simulink library "seriallib"  (Simulink 5.0)
undefined symbols (not defined in the file or in its folder): mbaseserialmask, mmodemcontrol, mquamask, mrs232
libraries: xpclib x193, vxlib x36, simulink x4
(part 1 of 3)
settings Model: Creator=gweast  LastModifiedBy=gweast

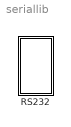
== system seriallib ==
  RS232 : Subsystem

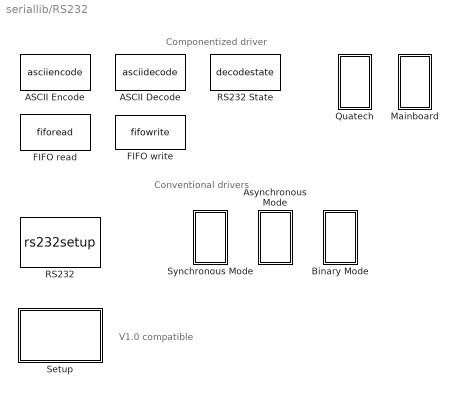
== system seriallib/RS232 ==
  note: Conventional drivers
  note: Componentized driver
  note: V1.0 compatible
  "ASCII Decode " : S-Function  FunctionName=asciidecode  Parameters=format, nvars, varids  mask(Asynchronous FIFO Block: reader){format=%d\r, nvars=1, vartypes={ }}
      mask prompts: format "Format string:"; nvars "Number of variables:"; vartypes "Variable types:"
      mask help: FIFO read
      mask init:
      | [ maskdisplay, varids, format ] = masciidecode( 2, format, nvars, vartypes, 1 );
      | set_param( gcb, 'MaskDisplay', maskdisplay );
      mask Help: helpview(fullfile(docroot, 'mapfiles', 'xpc.map'), 'Quatech_ASCII_Decode')
      mask Display: disp( 'ASCII\nDecode');port_label('input',1,'D');port_label('output',1,'1');
  "ASCII Encode " : S-Function  FunctionName=asciiencode  Parameters=format, maxlength, nvars, varids  mask(Ascii Encode){format=%d\r, nvars=1, maxlength=128, vartypes={ 'double' }}
      mask prompts: format "Format string:"; nvars "Number of variables:"; maxlength "Max output string length:"; vartypes "Variable types:"
      mask help: Ascii Encode -- encode input variables as ascii for RS232.
      mask init:
      | [ maskdisplay, varids, format ] = masciidecode( 2, format, nvars, vartypes, 2 );
      | set_param( gcb, 'MaskDisplay', maskdisplay );
      mask Help: helpview(fullfile(docroot, 'mapfiles', 'xpc.map'), 'Quatech_ASCII_Encode')
      mask Display: disp( 'ASCII\nEncode');port_label('output',1,'D');port_label('input',1,'1');
  Asynchronous Mode : Subsystem
  Binary Mode : Subsystem
  "FIFO read " : S-Function  FunctionName=fiforead  Parameters=maxsize, minsize, usedelimiter, delimiter, outputtype, sampletime, enable, enableout  mask(Asynchronous FIFO Block: reader){maxsize=1024, minsize=1, usedelimiter=on, delimiter=13, outputtype=8 bit uint null terminated, enable=off, enableout=off, sampletime=0.001}
      mask prompts: maxsize "Maximum read size:"; minsize "Minimum read size:"; usedelimiter "Read to delimiter:"; outputtype "Output vector type:"; enable "Max and Min read size ports:"; enableout "Enable passthrough:"
      mask help: FIFO read
      mask init:
      | maskdisplay = mfiforw( enable, enableout, 2 );
      | set_param( gcb, 'MaskDisplay', maskdisplay );
      mask Help: helpview(fullfile(docroot, 'mapfiles', 'xpc.map'), 'Quatech_FIFO_Read')
      mask StyleString: edit,edit,checkbox,edit,popup(count+32 bit int|count+32 bit uint|count+16 bit int|count+16 bit uint|8 bit int null terminated|8 bit uint null terminated),checkbox,checkbox,edit
      mask Display: disp( 'FIFO\nRead');port_label('output',1,'D');port_label('input',1,'F');
  "FIFO write " : S-Function  FunctionName=fifowrite  Parameters=size, inputtype, sampletime, present  mask(Asynchronous FIFO Block: writer){size=1024, inputtype=8 bit uint null terminated, present=off, sampletime=-1}
      mask prompts: inputtype "Input vector type:"; present "Data present output:"
      mask help: FIFO write
      mask init:
      | maskdisplay = mfiforw( present, 0, 1 );
      | set_param(gcb,'MaskDisplay',maskdisplay);
      mask Help: helpview(fullfile(docroot, 'mapfiles', 'xpc.map'), 'Quatech_FIFO_Write')
      mask StyleString: edit,popup(count+32 bit int|count+32 bit uint|count+16 bit int|count+16 bit uint|8 bit int null terminated|8 bit uint null terminated),checkbox,edit
      mask Display: disp( 'FIFO\nwrite');port_label('input',1,'D');port_label('output', 1, 'F');
  Mainboard : Subsystem
  Quatech : Subsystem
  "RS232 " : S-Function  InitFcn=mrs232(0);  FunctionName=rs232setup  Parameters=port, baud, dbits, sbits, parity, prot, sbuf, rbuf, 0, istr, iack, iackto, tstr, tack, tackto, initinfo, initackinfo, terminfo, termackinfo  mask(rs232setup){port=COM1, baud=9600, dbits=8, sbits=1, parity=None, prot=None, sbuf=1024, rbuf=1024, initstruct=[], termstruct=[]}
      mask prompts: baud "Baud rate:"; dbits "Number of data bits:"; sbits "Number of stop bits:"; prot "Protocol:"; sbuf "Send buffer size:"; rbuf "Receive buffer size:"; initstruct "Initialization command structure:"; termstruct "Termination command structure:"
      mask help:
      | RS-232
      | Mainboard
      | Setup
      mask init:
      | dmy = '';
      | [istr,iack,dmy,maskdisplay,maskdescription,dmy,dmy,dmy,dmy,initinfo,initackinfo,iackto]=mrs232(2,initstruct,4);
      | [tstr,tack,dmy,maskdisplay,maskdescription,dmy,dmy,dmy,dmy,terminfo,termackinfo,tackto]=mrs232(1,termstruct,4);
      | set_param(gcb,'MaskDisplay',maskdisplay);
      | set_param(gcb,'MaskDescription',maskdescription);
      mask Help: helpview(fullfile(docroot, 'mapfiles', 'xpc.map'), 'RS232_RS232')
      mask StyleString: popup(COM1|COM2|COM3|COM4),popup(115200|57600|38400|19200|9600|4800|2400|1200|600|300|110),popup(8|7),popup(1|2),popup(None|Odd|Even),popup(None|XOn XOff),edit,edit,edit,edit
      mask Display: disp('RS-232\nMainboard\nSetup');
  RS232 State : S-Function  FunctionName=decodestate  Parameters=overrun, parity, frame, breakint, count  mask(RS232 State){overrun=on, parity=on, frame=off, breakint=off}
      mask prompts: overrun "Overrun error output:"; parity "Parity error output"; frame "Framing error output"; breakint "Break interrupt output"
      mask help: RS232 State
      mask init:
      | count = 0;
      | [maskdisplay, count] = mdecodestate( overrun, parity, frame, breakint );
      | set_param( gcb, 'MaskDisplay', maskdisplay );
      mask Help: helpview(fullfile(docroot, 'mapfiles', 'xpc.map'), 'Quatech_State')
      mask Display: disp('RS232\nState');port_label('input',1,'D');port_label('output',1,'D');port_label('output',2,'O');port_label('output',3,'P');
  "Setup " : Subsystem  mask(rs232setup){port=COM2, baudrate=115200, databit=8, stopbit=1, parity=None, protocol=None, sendbuf=1024, recbuf=1024}
      mask prompts: baudrate "Baud rate:"; databit "Number of data bits:"; stopbit "Number of stop bits:"; sendbuf "Send buffer size:"; recbuf "Receive buffer size:"
      mask Help: helpview(fullfile(docroot,'mapfiles','xpc.map'),'RS232_Setup');
      mask StyleString: popup(COM1|COM2|COM3|COM4),popup(115200|57600|38400|19200|9600|4800|2400|1200|300|110),popup(8|7|6|5),popup(1|2),popup(None|Odd|Even),popup(None|XOnXOff|RTSCTS|DTRDSR),edit,edit
      mask Display: disp('RS232\nMainboard\nSetup');
  Synchronous Mode : Subsystem

== system seriallib/RS232/Asynchronous Mode ==
  note: V1.0 compatible
  "RS232 " : S-Function  FunctionName=rs232send  Parameters=port, inStr, inport, numinports, formatsendinfo, ts, waitarg  mask(rs232send){port=COM1, blockvar=[], ts=0.1}
      mask prompts: blockvar "Message struct name:"; ts "Sample time:"
      mask help:
      | RS-232
      | Mainboard
      | Send
      mask init:
      | inStr = '';
      | outStr = '';
      | [inStr,outStr,dtypes,maskdisplay,maskdescription,inport,outport, numinports, numoutports, formatsendinfo, formatrecinfo, waitarg] = mrs232 (1, blockvar, 2);
      | set_param(gcb,'MaskDisplay',maskdisplay);
      | set_param(gcb,'MaskDescription',maskdescription);
      mask Help: helpview(fullfile(docroot, 'mapfiles', 'xpc.map'), 'RS232_Asynchronous-Mode_RS232')
      mask StyleString: popup(COM1|COM2|COM3|COM4),edit,edit
      mask Display: disp('RS-232\nMainboard\nSend');
  RS232 1 : S-Function  FunctionName=rs232rec  Parameters=port, outStr, outport, numoutports, formatrecinfo, dtypes, ts, numeom  mask(rs232rec){port=COM1, blockvar=[], ts=0.1}
      mask prompts: blockvar "Message struct name:"; ts "Sample time:"
      mask help:
      | RS-232
      | Mainboard
      | Receive
      mask init:
      | inStr = '';
      | outStr = '';
      | [inStr,outStr,dtypes,maskdisplay,maskdescription,inport,outport, numinports, numoutports, formatsendinfo, formatrecinfo, waitarg, numeom] = mrs232 (1, blockvar, 1);
      | 
      | 
      | set_param(gcb,'MaskDisplay',maskdisplay);
      | set_param(gcb,'MaskDescription',maskdescription);
      mask Help: helpview(fullfile(docroot, 'mapfiles', 'xpc.map'), 'RS232_Asynchronous-Mode_RS232-1')
      mask StyleString: popup(COM1|COM2|COM3|COM4),edit,edit
      mask Display: disp('RS-232\nMainboard\nReceive');
  "Receive " : Subsystem  mask(rs232rec){port=COM2, formatrec='start,%f,stop;', numb=1, ts=0.01}
      mask prompts: formatrec "Receive format:"; numb "Number of end-of-message characters:"; ts "Sample time:"
      mask Help: helpview(fullfile(docroot, 'mapfiles', 'xpc.map'), 'RS232_Asynchronous-Mode_Receive')
      mask StyleString: popup(COM1|COM2|COM3|COM4),edit,edit,edit
      mask Display: disp('RS232\nMainboard\nReceive');
  "Send " : Subsystem  mask(rs232send){port=COM2, formatsend='start,%f,stop;', wait=off, ts=0.01}
      mask prompts: formatsend "Send format:"; wait "Wait until message is transmitted"; ts "Sample time:"
      mask Help: helpview(fullfile(docroot, 'mapfiles', 'xpc.map'), 'RS232_Asynchronous-Mode_Send')
      mask StyleString: popup(COM1|COM2|COM3|COM4),edit,checkbox,edit
      mask Display: disp('RS232\nMainboard\nSend');

== system seriallib/RS232/Binary Mode ==
  Pack : xpclib/UDP/Pack  datatypes={'double'}  byteAlign=1
  RS232 Binary Receive : S-Function  FunctionName=rs232brec  Parameters=port,width,samptime  mask(rs232brec){port=COM1, width=1, samptime=-1}
      mask prompts: port "COM port:"; width "Maximum width per packet:"; samptime "Sample time:"
      mask Help: helpview(fullfile(docroot, 'mapfiles', 'xpc.map'), 'RS232_Binary-Mode_RS232-Binary-Receive')
      mask StyleString: popup(COM1|COM2|COM3|COM4),edit,edit
      mask Display: port_label('input',  1, 'Length');port_label('input',  2, 'Enable');port_label('output', 1, 'Done');port_label('output', 2, 'Data');disp(sprintf('RS232 Receive\nCOM%d', port));
  RS232 Binary Send : S-Function  FunctionName=rs232bsend  Parameters=port,width,samptime  mask(rs232bsend){port=COM1, width=1, samptime=-1}
      mask prompts: port "COM port:"; width "Maximum width per packet:"; samptime "Sample time:"
      mask Help: helpview(fullfile(docroot, 'mapfiles', 'xpc.map'), 'RS232_Binary-Mode_RS232-Binary-Send')
      mask StyleString: popup(COM1|COM2|COM3|COM4),edit,edit
      mask Display: disp(sprintf('RS232 Send\nCOM%d', port));
  Unpack : xpclib/UDP/Unpack  dimensions={[1]}  datatypes={'double'}  byteAlign=1

== system seriallib/RS232/Mainboard ==
  Baseboard Serial : Subsystem  InitFcn=mbaseserialmask(4,2)  TreatAsAtomicUnit=on  mask(Baseboard RS232 Send Receive){group=Board Setup, port=1, irqnum=4, saddr1=0x3f8, saddr2=0x3e8, config=Com1/Com3, baud1=115200, parity1=None, ndata1=8, nstop1=1, fifomode1=16 deep, rlevel1=half full, automode1=on, xmtfifosize1=1024, xmtdatatype1=8 bit uint null terminated, rcvfifosize1=1024, rcvmaxread1=1024, rcvminread1=1, rcvusedelim1=on, rcvdelim1=13, rcvdatatype1=count+16 bit uint, rcvsampletime1=-1, baud2=115200, parity2=None, ndata2=8, nstop2=1, fifomode2=16 deep, rlevel2=half full, automode2=off, xmtfifosize2=1024, xmtdatatype2=8 bit uint null terminated, rcvfifosize2=1024, rcvmaxread2=1024, rcvminread2=1, rcvusedelim2=on, rcvdelim2=13, rcvdatatype2=count+16 bit uint, rcvsampletime2=-1}
      mask prompts: group "Parameter group:"; port "Port to modify:"; irqnum "IRQ number:"; saddr1 "First port address:"; saddr2 "Second port address:"; config "Configuration:"; baud1 "Baud rate:"; parity1 "Parity:"; ndata1 "Data bits:"; nstop1 "Stop bits:"; fifomode1 "Hardware fifo size:"; rlevel1 "Receive fifo interrupt level:"; automode1 "Auto RTS/CTS:"; xmtfifosize1 "Transmit software fifo size:"; xmtdatatype1 "Transmit fifo data type:"; rcvfifosize1 "Receive software fifo size:"; rcvmaxread1 "Receive maximum read:"; rcvminread1 "Receive minimum read:"; rcvusedelim1 "Read to delimiter:"; rcvdelim1 "Delimiter:"; rcvdatatype1 "Receive data type:"; rcvsampletime1 "Receive SampleTime:"; baud2 "Baud rate:"; parity2 "Parity:"; ndata2 "Data bits:"; nstop2 "Stop bits:"; fifomode2 "Hardware fifo size:"; rlevel2 "Receive fifo interrupt level:"; automode2 "Auto RTS/CTS:"; xmtfifosize2 "Transmit software fifo size:"; xmtdatatype2 "Transmit fifo data type:"; rcvfifosize2 "Receive software fifo size:"; rcvmaxread2 "Receive maximum read:"; rcvminread2 "Receive minimum read:"; rcvusedelim2 "Read to delimiter:"; rcvdelim2 "Delimiter:"; rcvdatatype2 "Receive data type:"; rcvsampletime2 "Receive SampleTime:"
      mask help:
      | Baseboard
      | RS232 Send Receive Subsystem
      mask init:
      | [addr1, addr2, maskdisplay] = mbaseserialmask( 1, 2 );
      | baddr1 = addr1;
      | baddr2 = addr2;
      | mbaseserialmask( 3, 2 );
      | set_param( gcb, 'MaskDisplay', maskdisplay );
      mask Help: helpview(fullfile(docroot, 'mapfiles', 'xpc.map'), 'Baseboard_Serial_Subsystem')
      mask StyleString: popup(Board Setup|Basic Setup|Transmit Setup|Receive Setup),popup(1|2),edit,edit,edit,popup(Com1/none|Com2/none|Com1/Com3|Com2/Com4|none/Com3|none/Com4|Custom),popup(921600|460800|230400|115200|57600|38400|19200|9600|4800|2400|1200|600|300|110),popup(None|Even|Odd|Mark|Space),popup(5|6|7|8),popup(1|2),popup(64 deep|16 deep|1 deep),popup(1|quarter full|half full|almost full),checkbox,edit,popup(count+32 bit int|count+32 bit uint|count+16 bit int|count+16 bit uint|8 bit int null terminated|8 bit uint null terminated),edit,edit,edit,checkbox,edit,popup(count+32 bit int|count+32 bit uint|count+16 bit int|count+16 bit uint|8 bit int null terminated|8 bit uint null terminated),edit,popup(921600|460800|230400|115200|57600|38400|19200|9600|4800|2400|1200|600|300|110),popup(None|Even|Odd|Mark|Space),popup(5|6|7|8),popup(1|2),popup(64 deep|16 deep|1 deep),popup(1|quarter full|half full|almost full),checkbox,edit,popup(count+32 bit int|count+32 bit uint|count+16 bit int|count+16 bit uint|8 bit int null terminated|8 bit uint null terminated),edit,edit,edit,checkbox,edit,popup(count+32 bit int|count+32 bit uint|count+16 bit int|count+16 bit uint|8 bit int null terminated|8 bit uint null terminated),edit
      mask CallbackString:
      | mbaseserialmask( 2, 2 );
      | |mbaseserialmask( 2, 2 );||||mbaseserialmask( 2, 2 );
      | ||||||||||||||||||||||||||||||||
      mask Display: disp('Baseboard\nRS232\nSend Receive')port_label('input',1,'XMT1');port_label('input',2,'XMT3');port_label('output',1,'RCV1');port_label('output',2,'RCV3');
  Baseboard Serial Internal  blocks : Subsystem
  Modem Control : S-Function  InitFcn=mmodemcontrol(4)  FunctionName=modemcontrolbase  Parameters=addr, boardtype, rts, dtr, count  mask(Baseboard Modem Control){rts=on, dtr=on, config=Com1, addr=0x3f8}
      mask prompts: config "Configuration:"; addr "Base address:"
      mask help:
      | Baseboard
      | Modem Control
      mask init:
      | count = 0;
      | boardtype = 4;
      | [maskdisplay, count, addr] = mmodemcontrol( 2, rts, dtr, boardtype, config, addr );
      | addr = hex2dec( addr(3:end) );
      | set_param( gcb, 'MaskDisplay', maskdisplay );
      mask Help: helpview(fullfile(docroot, 'mapfiles', 'xpc.map'), 'Baseboard_MODEM_Control')
      mask StyleString: checkbox,checkbox,popup(Com1|Com2|Com3|Com4|Custom),edit
      mask CallbackString:
      | ||mmodemcontrol( 1 );
      | |
      mask Display: disp('Baseboard\nModem Control');port_label('input',1,'RTS');port_label('input',2,'DTR');
  Modem Status : S-Function  FunctionName=modemstatusbase  Parameters=addr, boardtype, cts, dsr, ring, dcd, count, sampletime  mask(Modem Status){cts=on, dsr=on, ring=on, dcd=on, sampletime=-1, config=Com1, addr=0x3f8}
      mask prompts: ring "RI:"; config "Configuration:"; addr "Base address:"
      mask help:
      | Baseboard
      | Modem Status
      mask init:
      | count = 0;
      | boardtype = 4;
      | [maskdisplay, count, addr] = mmodemstatus( 2, cts, dsr, ring, dcd, boardtype, config, addr );
      | addr = hex2dec( addr(3:end) );
      | set_param( gcb, 'MaskDisplay', maskdisplay );
      mask Help: helpview(fullfile(docroot, 'mapfiles', 'xpc.map'), 'Baseboard_MODEM_Status')
      mask StyleString: checkbox,checkbox,checkbox,checkbox,edit,popup(Com1|Com2|Com3|Com4|Custom),edit
      mask CallbackString:
      | |||||mmodemstatus( 1 );
      | |
      mask Display: disp('Baseboard\nModem Status');port_label('output',1,'CTS');port_label('output',2,'DSR');port_label('output',3,'RI');port_label('output',4,'DCD');

== system seriallib/RS232/Quatech ==
  ESC-100 : Subsystem
  QSC-100 : Subsystem
  QSC-200/300 : Subsystem

== system seriallib/RS232/Setup  ==
  S-Function : S-Function  FunctionName=rs232_setup  Parameters=port,baudrate,databit, stopbit, parity, protocol, sendbuf, recbuf, 0

== system seriallib/RS232/Synchronous Mode ==
  note: V1.0 compatible
  "RS232 " : S-Function  FunctionName=rs232sendrec  Parameters=port, inStr, outStr, inport, outport, numinports, numoutports, formatsendinfo, formatrecinfo, waitarg, dtypes, ts, numeom, timeoutarg  mask(rs232sendrec){port=COM1, blockvar=[], ts=0.1}
      mask prompts: blockvar "Message struct name:"; ts "Sample time:"
      mask help:
      | RS-232
      | Mainboard
      | Send/Receive
      mask init:
      | inStr = '';
      | outStr = '';
      | [inStr,outStr,dtypes,maskdisplay,maskdescription,inport,outport, numinports, numoutports, formatsendinfo, formatrecinfo, waitarg, numeom, timeoutarg] = mrs232 (1, blockvar, 3);
      | set_param(gcb,'MaskDisplay',maskdisplay);
      | set_param(gcb,'MaskDescription',maskdescription);
      mask Help: helpview(fullfile(docroot, 'mapfiles', 'xpc.map'), 'RS232_Synchronous-Mode_RS232')
      mask StyleString: popup(COM1|COM2|COM3|COM4),edit,edit
      mask Display: disp('RS-232\nMainboard\nSend/Receive');
  "Send & Receive " : Subsystem  mask(rs232sendrec){port=COM2, formatsend='start,%f,stop;', formatrec='start,%f,stop;', numb=1, ts=0.01}
      mask prompts: formatsend "Send format:"; formatrec "Receive format:"; numb "Number of end-of-message characters:"; ts "Sample time:"
      mask Help: helpview(fullfile(docroot, 'mapfiles', 'xpc.map'), 'RS232_Synchronous-Mode_Send-&-Receive')
      mask StyleString: popup(COM1|COM2|COM3|COM4),edit,edit,edit,edit
      mask Display: disp('RS232\nMainboard\nSend/Receive');

== system seriallib/RS232/Asynchronous Mode/Receive  ==
  S-Function : S-Function  FunctionName=rs232_rec  Parameters=port,formatrec,numb,ts
  Out1 : Outport
  wires:
  S-Function/1 -> Out1/1

== system seriallib/RS232/Asynchronous Mode/Send  ==
  In1 : Inport
  S-Function : S-Function  FunctionName=rs232_send  Parameters=port,formatsend,wait,ts
  wires:
  In1/1 -> S-Function/1

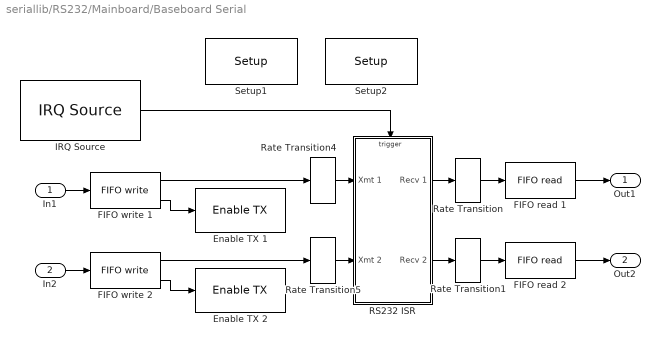
== system seriallib/RS232/Mainboard/Baseboard Serial ==
  In1 : Inport
  In2 : Inport  Port=2
  Enable TX 1 : xpclib/RS232/Mainboard/Baseboard Serial Internal  blocks/Enable TX   addr=baddr1
  Enable TX 2 : xpclib/RS232/Mainboard/Baseboard Serial Internal  blocks/Enable TX   addr=baddr2
  FIFO read 1 : xpclib/RS232/FIFO read   maxsize=1024  minsize=1  usedelimiter=on  delimiter=13  outputtype=count+16 bit uint  enable=off  enableout=off  sampletime=-1
  FIFO read 2 : xpclib/RS232/FIFO read   maxsize=1024  minsize=1  usedelimiter=on  delimiter=13  outputtype=count+16 bit uint  enable=off  enableout=off  sampletime=-1
  FIFO write 1 : xpclib/RS232/FIFO write   size=1024  inputtype=8 bit uint null terminated  present=on  sampletime=-1
  FIFO write 2 : xpclib/RS232/FIFO write   size=1024  inputtype=8 bit uint null terminated  present=on  sampletime=-1
  IRQ Source : xpclib/Asynchronous Event/IRQ Source  irqNo=4  preempt=off  b_type=None/Other  slot=-1
  RS232 ISR : Subsystem  TreatAsAtomicUnit=on  mask(RS232 ISR){addr1=baddr1, addr2=baddr2}
      mask prompts: addr1 "First channel address:"; addr2 "Second channel address:"
      mask help:
      | Baseboard Serial
      | Interrupt Service Routine
      mask init:
      | baddr1 = addr1;
      | baddr2 = addr2;
      mask Display:
      | disp('Baseboard\nSerial\nISR');
      | port_label('input', 1, 'XMT1');
      | port_label('input', 2, 'XMT3');
      | port_label('output', 1, 'RCV1');
      | port_label('output', 2, 'RCV3');
  Rate Transition{,1,4..5} (4 alike) : vxlib/Asynchronous Support/Rate Transition  sample_time=-1
  Setup1 : xpclib/RS232/Mainboard/Baseboard Serial Internal  blocks/Setup  baud=115200  width=8  nstop=1  parity=None  fmode=16 deep  rlevel=half full  ctsmode=on  addr=baddr1
  Setup2 : xpclib/RS232/Mainboard/Baseboard Serial Internal  blocks/Setup  baud=115200  width=8  nstop=1  parity=None  fmode=16 deep  rlevel=half full  ctsmode=off  addr=baddr2
  Out1 : Outport
  Out2 : Outport  Port=2
  wires:
  FIFO write 1/2 -> Enable TX 1/1
  IRQ Source/1 -> RS232 ISR/Trigger
  Rate Transition4/1 -> RS232 ISR/1(Xmt 1)
  RS232 ISR/1(Recv 1) -> Rate Transition/1
  RS232 ISR/2(Recv 2) -> Rate Transition1/1
  FIFO write 1/1 -> Rate Transition4/1
  In1/1 -> FIFO write 1/1
  FIFO write 2/1 -> Rate Transition5/1
  In2/1 -> FIFO write 2/1
  Rate Transition/1 -> FIFO read 1/1
  FIFO read 1/1 -> Out1/1
  Rate Transition1/1 -> FIFO read 2/1
  FIFO read 2/1 -> Out2/1
  FIFO write 2/2 -> Enable TX 2/1
  Rate Transition5/1 -> RS232 ISR/2(Xmt 2)

== system seriallib/RS232/Mainboard/Baseboard Serial Internal  blocks ==
  "Enable TX " : S-Function  FunctionName=sertxenablebase  Parameters=addr  mask(Enable TX Int){addr=0}
      mask prompts: addr "Base address:"
      mask help:
      | Baseboard Serial
      | Enable TX Interrupt
      mask init:
      | addr = hex2dec( addr(3:end) );
      mask Help: helpview(fullfile(docroot, 'mapfiles', 'xpc.map'), 'Baseboard_Enable_Int')
      mask Display:
      | disp('Baseboard\nSerial\nEnable TX Int');
      | port_label('input', 1, 'E');
  Filter Int Reason : S-Function  FunctionName=filterserint  Parameters=port, value  mask(Interrupt Source Filter){port=1, value=Receive data}
      mask prompts: value "Filter value:"
      mask help:
      | Baseboard
      | Interrupt Source Filter
      mask Help: helpview(fullfile(docroot, 'mapfiles', 'xpc.map'), 'Baseboard_Filter_Ints')
      mask StyleString: popup(1|2),popup(Receive data|Transmitter empty|Modem status change)
      mask Display:
      | disp('Baseboard\nSerial\nFilter Int Reason');
      | port_label('input', 1, 'S' );
      | port_label('output', 1, 'E' );
  Read HW FIFO : S-Function  FunctionName=serreadbase  Parameters=addr, flush  mask(Read Data Port){flush=on, addr=0}
      mask prompts: flush "Flush HW FIFO on startup"; addr "Base address:"
      mask help:
      | Baseboard
      | Read Data Port
      mask init:
      | addr = hex2dec( addr(3:end) );
      mask Help: helpview(fullfile(docroot, 'mapfiles', 'xpc.map'), 'Baseboard_Read_HW')
      mask Display:
      | disp('Baseboard\nSerial\nRead HW FIFO');
      | port_label('input', 1, 'E');
      | port_label('output', 1, 'D');
  Read Int Status : S-Function  FunctionName=Iquerybase  Parameters=addr1, addr2  mask(Interrupt Query){addr1=0, addr2=0}
      mask prompts: addr1 "Base address 1"; addr2 "Base address 2"
      mask help:
      | Baseboard Serial
      | Interrupt Query
      mask init:
      | addr1 = hex2dec( addr1(3:end) );
      | addr2 = hex2dec( addr2(3:end) );
      mask Help: helpview(fullfile(docroot, 'mapfiles', 'xpc.map'), 'Baseboard_Interrupt_Query')
      mask Display:
      | disp('Baseboard\nSerial\nRead Int Status');
      | port_label('output', 1, 'S' );
  Setup : S-Function  FunctionName=sersetupbase  Parameters=addr, baud, width, nstop, parity, fmode, ctsmode, rlevel  mask(setup){baud=115200, width=8, nstop=1, parity=None, fmode=16 deep, rlevel=half full, ctsmode=off, addr=0}
      mask prompts: baud "Baud rate:"; width "Number of data bits:"; nstop "Number of stop bits:"; fmode "Fifo mode:"; rlevel "Receive trigger level:"; ctsmode "Enable auto RTS/CTS"; addr "Base Address:"
      mask help:
      | Baseboard
      | Serial
      | Setup
      mask init:
      | addr = hex2dec( addr(3:end) );
      mask Help: helpview(fullfile(docroot, 'mapfiles', 'xpc.map'), 'Baseboard_Setup')
      mask StyleString: popup(115200|57600|38400|19200|9600|4800|2400|1200|600|300|110),popup(5|6|7|8),popup(1|2),popup(None|Even|Odd|Mark|Space),popup(64 deep|16 deep|1 deep),popup(1|quarter full|half full|almost full),checkbox,edit
      mask Display: disp('Baseboard\nSerial\nSetup');
  Write HW FIFO : S-Function  FunctionName=serwritebase  Parameters=addr  mask(Write Data Port){addr=0}
      mask prompts: addr "Base address:"
      mask help:
      | Baseboard
      | Write Data Port
      mask init:
      | addr = hex2dec( addr(3:end) );
      mask Help: helpview(fullfile(docroot, 'mapfiles', 'xpc.map'), 'Baseboard_Write_HW')
      mask Display:
      | disp('Baseboard\nSerial\nWrite HW FIFO');
      | port_label('input', 1, 'D');
      | port_label('input', 2, 'E');

== system seriallib/RS232/Quatech/ESC-100 ==
  ESC-100 : Subsystem  InitFcn=mquamask(3)  TreatAsAtomicUnit=on  mask(ESC-100 RS232 Send Receive){group=Board Setup, port=1, irqnum=7, slot=-1, baud1=19200, parity1=None, ndata1=8, nstop1=1, fifomode1=64 deep, rlevel1=half full, automode1=on, xmtfifosize1=1024, xmtdatatype1=8 bit uint null terminated, rcvfifosize1=1024, rcvmaxread1=1024, rcvminread1=1, rcvusedelim1=on, rcvdelim1=13, rcvdatatype1=count+16 bit uint, rcvsampletime1=-1, baud2=19200, parity2=None, ndata2=8, nstop2=1, fifomode2=64 deep, rlevel2=half full, automode2=on, xmtfifosize2=1024, xmtdatatype2=8 bit uint null terminated, rcvfifosize2=1024, rcvmaxread2=1024, rcvminread2=1, rcvusedelim2=on, rcvdelim2=13, rcvdatatype2=count+16 bit uint, rcvsampletime2=-1, baud3=19200, parity3=None, ndata3=8, nstop3=1, fifomode3=64 deep, rlevel3=half full, automode3=on, xmtfifosize3=1024, xmtdatatype3=8 bit uint null terminated, rcvfifosize3=1024, rcvmaxread3=1024, rcvminread3=1, rcvusedelim3=on, rcvdelim3=13, rcvdatatype3=count+16 bit uint, rcvsampletime3=-1, buad4=19200, parity4=None, ndata4=8, nstop4=1, fifomode4=64 deep, rlevel4=half full, automode4=on, xmtfifosize4=1024, xmtdatatype4=8 bit uint null terminated, rcvfifosize4=1024, rcvmaxread4=1024, rcvminread4=1, rcvusedelim4=on, rcvdelim4=13, rcvdatatype4=count+16 bit uint, rcvsampletime4=-1, baud5=19200, parity5=None, ndata5=8, nstop5=1, fifomode5=64 deep, rlevel5=half full, automode5=on, xmtfifosize5=1024, xmtdatatype5=8 bit uint null terminated, rcvfifosize5=1024, rcvmaxread5=1024, rcvminread5=1, rcvusedelim5=on, rcvdelim5=13, rcvdatatype5=count+16 bit uint, rcvsampletime5=-1, baud6=19200, parity6=None, ndata6=8, nstop6=1, fifomode6=64 deep, rlevel6=half full, automode6=on, xmtfifosize6=1024, xmtdatatype6=8 bit uint null terminated, rcvfifosize6=1024, rcvmaxread6=1024, rcvminread6=1, rcvusedelim6=on, rcvdelim6=13, rcvdatatype6=count+16 bit uint, rcvsampletime6=-1, baud7=19200, parity7=None, ndata7=8, nstop7=1, fifomode7=64 deep, rlevel7=half full, automode7=on, xmtfifosize7=1024, xmtdatatype7=8 bit uint null terminated, rcvfifosize7=1024, rcvmaxread7=1024, rcvminread7=1, rcvusedelim7=on, rcvdelim7=13, rcvdatatype7=count+16 bit uint, rcvsampletime7=-1, baud8=19200, parity8=None, ndata8=8, nstop8=1, fifomode8=64 deep, rlevel8=half full, automode8=on, xmtfifosize8=1024, xmtdatatype8=8 bit uint null terminated, rcvfifosize8=1024, rcvmaxread8=1024, rcvminread8=1, rcvusedelim8=on, rcvdelim8=13, rcvdatatype8=count+16 bit uint, rcvsampletime8=-1}
      mask prompts: group "Parameter group:"; port "Port to modify:"; irqnum "IRQ number:"; baud1 "Baud rate:"; parity1 "Parity:"; ndata1 "Data bits:"; nstop1 "Stop bits:"; fifomode1 "Hardware fifo size:"; rlevel1 "Receive fifo interrupt level:"; automode1 "Auto RTS/CTS:"; xmtfifosize1 "Transmit software fifo size:"; xmtdatatype1 "Transmit fifo data type:"; rcvfifosize1 "Receive software fifo size:"; rcvmaxread1 "Receive maximum read:"; rcvminread1 "Receive minimum read:"; rcvusedelim1 "Read to delimiter:"; rcvdelim1 "Delimiter:"; rcvdatatype1 "Receive data type:"; rcvsampletime1 "Receive SampleTime:"; baud2 "Baud rate:"; parity2 "Parity:"; ndata2 "Data bits:"; nstop2 "Stop bits:"; fifomode2 "Hardware fifo size:"; rlevel2 "Receive fifo interrupt level:"; automode2 "Auto RTS/CTS:"; xmtfifosize2 "Transmit software fifo size:"; xmtdatatype2 "Transmit fifo data type:"; rcvfifosize2 "Receive software fifo size:"; rcvmaxread2 "Receive maximum read:"; rcvminread2 "Receive minimum read:"; rcvusedelim2 "Read to delimiter:"; rcvdelim2 "Delimiter:"; rcvdatatype2 "Receive data type:"; rcvsampletime2 "Receive SampleTime:"; baud3 "Baud rate:"; parity3 "Parity:"; ndata3 "Data bits:"; nstop3 "Stop bits:"; fifomode3 "Hardware fifo size:"; rlevel3 "Receive fifo interrupt level:"; automode3 "Auto RTS/CTS:"; xmtfifosize3 "Transmit software fifo size:"; xmtdatatype3 "Transmit fifo data type:"; rcvfifosize3 "Receive software fifo size:"; rcvmaxread3 "Receive maximum read:"; rcvminread3 "Receive minimum read:"; rcvusedelim3 "Read to delimiter:"; rcvdelim3 "Delimiter:"; rcvdatatype3 "Receive data type:"; rcvsampletime3 "Receive SampleTime:"; buad4 "Baud rate:"; parity4 "Parity:"; ndata4 "Data bits:"; nstop4 "Stop bits:"; fifomode4 "Hardware fifo size:"; rlevel4 "Receive fifo interrupt level:"; automode4 "Auto RTS/CTS:"; xmtfifosize4 "Transmit software fifo size:"; xmtdatatype4 "Transmit fifo data type:"; rcvfifosize4 "Receive software fifo size:"; rcvmaxread4 "Receive maximum read:"; rcvminread4 "Receive minimum read:"; rcvusedelim4 "Read to delimiter:"; rcvdelim4 "Delimiter:"; rcvdatatype4 "Receive data type:"; rcvsampletime4 "Receive SampleTime:"; baud5 "Baud rate:"; parity5 "Parity:"; ndata5 "Data bits:"; nstop5 "Stop bits:"; fifomode5 "Hardware fifo size:"; rlevel5 "Receive fifo interrupt level:"; automode5 "Auto RTS/CTS:"; xmtfifosize5 "Transmit software fifo size:"; xmtdatatype5 "Transmit fifo data type:"; rcvfifosize5 "Receive software fifo size:"; rcvmaxread5 "Receive maximum read:"; rcvminread5 "Receive minimum read:"; rcvusedelim5 "Read to delimiter:"; rcvdelim5 "Delimiter:"; rcvdatatype5 "Receive data type:"; rcvsampletime5 "Receive SampleTime:"; baud6 "Baud rate:"; parity6 "Parity:"; ndata6 "Data bits:"; nstop6 "Stop bits:"; fifomode6 "Hardware fifo size:"; rlevel6 "Receive fifo interrupt level:"; automode6 "Auto RTS/CTS:"; xmtfifosize6 "Transmit software fifo size:"; xmtdatatype6 "Transmit fifo data type:"; rcvfifosize6 "Receive software fifo size:"; rcvmaxread6 "Receive maximum read:"; rcvminread6 "Receive minimum read:"; rcvusedelim6 "Read to delimiter:"; rcvdelim6 "Delimiter:"; rcvdatatype6 "Receive data type:"; rcvsampletime6 "Receive SampleTime:"; baud7 "Baud rate:"; parity7 "Parity:"; ndata7 "Data bits:"; nstop7 "Stop bits:"; fifomode7 "Hardware fifo size:"; rlevel7 "Receive fifo interrupt level:"; automode7 "Auto RTS/CTS:"; xmtfifosize7 "Transmit software fifo size:"; xmtdatatype7 "Transmit fifo data type:"; rcvfifosize7 "Receive software fifo size:"; rcvmaxread7 "Receive maximum read:"; rcvminread7 "Receive minimum read:"; rcvusedelim7 "Read to delimiter:"; rcvdelim7 "Delimiter:"; rcvdatatype7 "Receive data type:"; rcvsampletime7 "Receive SampleTime:"; baud8 "Baud rate:"; parity8 "Parity:"; ndata8 "Data bits:"; nstop8 "Stop bits:"; fifomode8 "Hardware fifo size:"; rlevel8 "Receive fifo interrupt level:"; automode8 "Auto RTS/CTS:"; xmtfifosize8 "Transmit software fifo size:"; xmtdatatype8 "Transmit fifo data type:"; rcvfifosize8 "Receive software fifo size:"; rcvmaxread8 "Receive maximum read:"; rcvminread8 "Receive minimum read:"; rcvusedelim8 "Read to delimiter:"; rcvdelim8 "Delimiter:"; rcvdatatype8 "Receive data type:"; rcvsampletime8 "Receive SampleTime:"
      mask help:
      | ESC-100
      | Quatech
      | RS232 Send Receive Subsystem
      mask init:
      | brdslot = slot;
      | mquamask( 1, 8 );
      mask Help: helpview(fullfile(docroot, 'mapfiles', 'xpc.map'), 'Quatech_Subsystem')
      mask StyleString: popup(Board Setup|Basic Setup|Transmit Setup|Receive Setup),popup(1|2|3|4|5|6|7|8),edit,edit,popup(921600|460800|230400|115200|57600|38400|19200|9600|4800|2400|1200|600|300|110),popup(None|Even|Odd|Mark|Space),popup(5|6|7|8),popup(1|2),popup(64 deep|16 deep|1 deep),popup(1|quarter full|half full|almost full),checkbox,edit,popup(count+32 bit int|count+32 bit uint|count+16 bit int|count+16 bit uint|8 bit int null terminated|8 bit uint null terminated),edit,edit,edit,checkbox,edit,popup(count+32 bit int|count+32 bit uint|count+16 bit int|count+16 bit uint|8 bit int null terminated|8 bit uint null terminated),edit,popup(921600|460800|230400|115200|57600|38400|19200|9600|4800|2400|1200|600|300|110),popup(None|Even|Odd|Mark|Space),popup(5|6|7|8),popup(1|2),popup(64 deep|16 deep|1 deep),popup(1|quarter full|half full|almost full),checkbox,edit,popup(count+32 bit int|count+32 bit uint|count+16 bit int|count+16 bit uint|8 bit int null terminated|8 bit uint null terminated),edit,edit,edit,checkbox,edit,popup(count+32 bit int|count+32 bit uint|count+16 bit int|count+16 bit uint|8 bit int null terminated|8 bit uint null terminated),edit,popup(921600|460800|230400|115200|57600|38400|19200|9600|4800|2400|1200|600|300|110),popup(None|Even|Odd|Mark|Space),popup(5|6|7|8),popup(1|2),popup(64 deep|16 deep|1 deep),popup(1|quarter full|half full|almost full),checkbox,edit,popup(count+32 bit int|count+32 bit uint|count+16 bit int|count+16 bit uint|8 bit int null terminated|8 bit uint null terminated),edit,edit,edit,checkbox,edit,popup(count+32 bit int|count+32 bit uint|count+16 bit int|count+16 bit uint|8 bit int null terminated|8 bit uint null terminated),edit,popup(921600|460800|230400|115200|57600|38400|19200|9600|4800|2400|1200|600|300|110),popup(None|Even|Odd|Mark|Space),popup(5|6|7|8),popup(1|2),popup(64 deep|16 deep|1 deep),popup(1|quarter full|half full|almost full),checkbox,edit,popup(count+32 bit int|count+32 bit uint|count+16 bit int|count+16 bit uint|8 bit int null terminated|8 bit uint null terminated),edit,edit,edit,checkbox,edit,popup(count+32 bit int|count+32 bit uint|count+16 bit int|count+16 bit uint|8 bit int null terminated|8 bit uint null terminated),edit,popup(921600|460800|230400|115200|57600|38400|19200|9600|4800|2400|1200|600|300|110),popup(None|Even|Odd|Mark|Space),popup(5|6|7|8),popup(1|2),popup(64 deep|16 deep|1 deep),popup(1|quarter full|half full|almost full),checkbox,edit,popup(count+32 bit int|count+32 bit uint|count+16 bit int|count+16 bit uint|8 bit int null terminated|8 bit uint null terminated),edit,edit,edit,checkbox,edit,popup(count+32 bit int|count+32 bit uint|count+16 bit int|count+16 bit uint|8 bit int null terminated|8 bit uint null terminated),edit,popup(921600|460800|230400|115200|57600|38400|19200|9600|4800|2400|1200|600|300|110),popup(None|Even|Odd|Mark|Space),popup(5|6|7|8),popup(1|2),popup(64 deep|16 deep|1 deep),popup(1|quarter full|half full|almost full),checkbox,edit,popup(count+32 bit int|count+32 bit uint|count+16 bit int|count+16 bit uint|8 bit int null terminated|8 bit uint null terminated),edit,edit,edit,checkbox,edit,popup(count+32 bit int|count+32 bit uint|count+16 bit int|count+16 bit uint|8 bit int null terminated|8 bit uint null terminated),edit,popup(921600|460800|230400|115200|57600|38400|19200|9600|4800|2400|1200|600|300|110),popup(None|Even|Odd|Mark|Space),popup(5|6|7|8),popup(1|2),popup(64 deep|16 deep|1 deep),popup(1|quarter full|half full|almost full),checkbox,edit,popup(count+32 bit int|count+32 bit uint|count+16 bit int|count+16 bit uint|8 bit int null terminated|8 bit uint null terminated),edit,edit,edit,checkbox,edit,popup(count+32 bit int|count+32 bit uint|count+16 bit int|count+16 bit uint|8 bit int null terminated|8 bit uint null terminated),edit,popup(921600|460800|230400|115200|57600|38400|19200|9600|4800|2400|1200|600|300|110),popup(None|Even|Odd|Mark|Space),popup(5|6|7|8),popup(1|2),popup(64 deep|16 deep|1 deep),popup(1|quarter full|half full|almost full),checkbox,edit,popup(count+32 bit int|count+32 bit uint|count+16 bit int|count+16 bit uint|8 bit int null terminated|8 bit uint null terminated),edit,edit,edit,checkbox,edit,popup(count+32 bit int|count+32 bit uint|count+16 bit int|count+16 bit uint|8 bit int null terminated|8 bit uint null terminated),edit
      mask CallbackString:
      | mquamask( 2, 8 );
      | |mquamask( 2, 8 );||||||||||||||||||||||||||||||||||||||||||||||||||||||||||||||||||||||||||||||||||||||||||||||||||||||||||||||||||||||||||||||||||
      mask Display:
      | disp('ESC-100\n\nRS232\n\nSend Receive');
      | port_label( 'input', 1, 'XMT1' );
      | port_label( 'input', 2, 'XMT2' );
      | port_label( 'input', 3, 'XMT3' );
      | port_label( 'input', 4, 'XMT4' );
      | port_label( 'input', 5, 'XMT5' );
      | port_label( 'input', 6, 'XMT6' );
      | port_label( 'input', 7, 'XMT7' );
      | port_label( 'input', 8, 'XMT8' );
      | port_label( 'output', 1, 'RCV1' );
      | port_label( 'output', 2, 'RCV2' );
      | port_label( 'output', 3, 'RCV3' );
      | port_label( 'output', 4, 'RCV4' );
      | port_label( 'output', 5, 'RCV5' );
      | port_label( 'output', 6, 'RCV6' );
      | port_label( 'output', 7, 'RCV7' );
      | port_label( 'output', 8, 'RCV8' );
  ESC-100 Internal blocks : Subsystem
  Modem Control : S-Function  InitFcn=mmodemcontrol(3)  FunctionName=modemcontrolqua  Parameters=slot, port, boardtype, rts, dtr, count  mask(ESC-100 Modem Control){port=1, rts=on, dtr=on, slot=-1}
      mask prompts: slot "PCI slot: (-1 for autosearch)"
      mask help:
      | ESC-100
      | Quatech
      | Modem Control
      mask init:
      | count = 0;
      | boardtype = 2;
      | [maskdisplay, count] = mmodemcontrol( 2, rts, dtr, boardtype, 0, 0 );
      | set_param( gcb, 'MaskDisplay', maskdisplay );
      mask Help: helpview(fullfile(docroot, 'mapfiles', 'xpc.map'), 'Quatech_MODEM_Control')
      mask StyleString: popup(1|2|3|4|5|6|7|8),checkbox,checkbox,edit
      mask Display: disp('ESC-100\nQuatech\nModem Control');port_label('input',1,'RTS');port_label('input',2,'DTR');
  Modem Status : S-Function  FunctionName=modemstatusqua  Parameters=slot, port, boardtype, cts, dsr, ring, dcd, count, sampletime  mask(Modem Status){port=1, cts=on, dsr=on, ring=on, dcd=on, sampletime=-1, slot=-1}
      mask prompts: ring "RI:"; slot "PCI slot: (-1 for autosearch)"
      mask help:
      | ESC-100
      | Quatech
      | Modem Status
      mask init:
      | count = 0;
      | boardtype = 2;
      | [maskdisplay, count] = mmodemstatus( 2, cts, dsr, ring, dcd, boardtype );
      | set_param( gcb, 'MaskDisplay', maskdisplay );
      mask Help: helpview(fullfile(docroot, 'mapfiles', 'xpc.map'), 'Quatech_MODEM_Status')
      mask StyleString: popup(1|2|3|4|5|6|7|8),checkbox,checkbox,checkbox,checkbox,edit,edit
      mask Display: disp('ESC-100\nQuatech\nModem Status');port_label('output',1,'CTS');port_label('output',2,'DSR');port_label('output',3,'RI');port_label('output',4,'DCD');

== system seriallib/RS232/Quatech/QSC-100 ==
  Modem Control : S-Function  InitFcn=mmodemcontrol(3)  FunctionName=modemcontrolqua  Parameters=slot, port, boardtype, rts, dtr, count  mask(QSC-100 Modem Control){port=1, rts=on, dtr=on, slot=-1}
      mask prompts: slot "PCI slot: (-1 for autosearch)"
      mask help:
      | QSC-100
      | Quatech
      | Modem Control
      mask init:
      | count = 0;
      | boardtype = 1;
      | [maskdisplay, count] = mmodemcontrol( 2, rts, dtr, boardtype, 0, 0 );
      | set_param( gcb, 'MaskDisplay', maskdisplay );
      mask Help: helpview(fullfile(docroot, 'mapfiles', 'xpc.map'), 'Quatech_MODEM_Control')
      mask StyleString: popup(1|2|3|4),checkbox,checkbox,edit
      mask Display: disp('QSC-100\nQuatech\nModem Control');port_label('input',1,'RTS');port_label('input',2,'DTR');
  Modem Status : S-Function  FunctionName=modemstatusqua  Parameters=slot, port, boardtype, cts, dsr, ring, dcd, count, sampletime  mask(Modem Status){port=1, cts=on, dsr=on, ring=on, dcd=on, sampletime=-1, slot=-1}
      mask prompts: ring "RI:"; slot "PCI slot: (-1 for autosearch)"
      mask help:
      | QSC-100
      | Quatech
      | Modem Status
      mask init:
      | count = 0;
      | boardtype = 1;
      | [maskdisplay, count] = mmodemstatus( 2, cts, dsr, ring, dcd, boardtype );
      | set_param( gcb, 'MaskDisplay', maskdisplay );
      mask Help: helpview(fullfile(docroot, 'mapfiles', 'xpc.map'), 'Quatech_MODEM_Status')
      mask StyleString: popup(1|2|3|4),checkbox,checkbox,checkbox,checkbox,edit,edit
      mask Display: disp('QSC-100\nQuatech\nModem Status');port_label('output',1,'CTS');port_label('output',2,'DSR');port_label('output',3,'RI');port_label('output',4,'DCD');
  QSC-100 : Subsystem  InitFcn=mquamask(3)  TreatAsAtomicUnit=on  mask(QSC-100 RS232 Send Receive){group=Transmit Setup, port=1, irqnum=7, slot=-1, baud1=115200, parity1=None, ndata1=8, nstop1=1, fifomode1=64 deep, rlevel1=half full, automode1=on, xmtfifosize1=1024, xmtdatatype1=8 bit uint null terminated, rcvfifosize1=1024, rcvmaxread1=1024, rcvminread1=1, rcvusedelim1=on, rcvdelim1=13, rcvdatatype1=count+16 bit uint, rcvsampletime1=-1, baud2=115200, parity2=None, ndata2=8, nstop2=1, fifomode2=64 deep, rlevel2=half full, automode2=on, xmtfifosize2=1024, xmtdatatype2=8 bit uint null terminated, rcvfifosize2=1024, rcvmaxread2=1024, rcvminread2=1, rcvusedelim2=on, rcvdelim2=13, rcvdatatype2=count+16 bit uint, rcvsampletime2=-1, baud3=115200, parity3=None, ndata3=8, nstop3=1, fifomode3=64 deep, rlevel3=half full, automode3=on, xmtfifosize3=1024, xmtdatatype3=8 bit uint null terminated, rcvfifosize3=1024, rcvmaxread3=1024, rcvminread3=1, rcvusedelim3=on, rcvdelim3=13, rcvdatatype3=count+16 bit uint, rcvsampletime3=-1, buad4=115200, parity4=None, ndata4=8, nstop4=1, fifomode4=64 deep, rlevel4=half full, automode4=on, xmtfifosize4=1024, xmtdatatype4=8 bit uint null terminated, rcvfifosize4=1024, rcvmaxread4=1024, rcvminread4=1, rcvusedelim4=on, rcvdelim4=13, rcvdatatype4=count+16 bit uint, rcvsampletime4=-1}
      mask prompts: group "Parameter group:"; port "Port to modify:"; irqnum "IRQ number:"; baud1 "Baud rate:"; parity1 "Parity:"; ndata1 "Data bits:"; nstop1 "Stop bits:"; fifomode1 "Hardware fifo size:"; rlevel1 "Receive fifo interrupt level:"; automode1 "Auto RTS/CTS:"; xmtfifosize1 "Transmit software fifo size:"; xmtdatatype1 "Transmit fifo data type:"; rcvfifosize1 "Receive software fifo size:"; rcvmaxread1 "Receive maximum read:"; rcvminread1 "Receive minimum read:"; rcvusedelim1 "Read to delimiter:"; rcvdelim1 "Delimiter:"; rcvdatatype1 "Receive data type:"; rcvsampletime1 "Receive SampleTime:"; baud2 "Baud rate:"; parity2 "Parity:"; ndata2 "Data bits:"; nstop2 "Stop bits:"; fifomode2 "Hardware fifo size:"; rlevel2 "Receive fifo interrupt level:"; automode2 "Auto RTS/CTS:"; xmtfifosize2 "Transmit software fifo size:"; xmtdatatype2 "Transmit fifo data type:"; rcvfifosize2 "Receive software fifo size:"; rcvmaxread2 "Receive maximum read:"; rcvminread2 "Receive minimum read:"; rcvusedelim2 "Read to delimiter:"; rcvdelim2 "Delimiter:"; rcvdatatype2 "Receive data type:"; rcvsampletime2 "Receive SampleTime:"; baud3 "Baud rate:"; parity3 "Parity:"; ndata3 "Data bits:"; nstop3 "Stop bits:"; fifomode3 "Hardware fifo size:"; rlevel3 "Receive fifo interrupt level:"; automode3 "Auto RTS/CTS:"; xmtfifosize3 "Transmit software fifo size:"; xmtdatatype3 "Transmit fifo data type:"; rcvfifosize3 "Receive software fifo size:"; rcvmaxread3 "Receive maximum read:"; rcvminread3 "Receive minimum read:"; rcvusedelim3 "Read to delimiter:"; rcvdelim3 "Delimiter:"; rcvdatatype3 "Receive data type:"; rcvsampletime3 "Receive SampleTime:"; buad4 "Baud rate:"; parity4 "Parity:"; ndata4 "Data bits:"; nstop4 "Stop bits:"; fifomode4 "Hardware fifo size:"; rlevel4 "Receive fifo interrupt level:"; automode4 "Auto RTS/CTS:"; xmtfifosize4 "Transmit software fifo size:"; xmtdatatype4 "Transmit fifo data type:"; rcvfifosize4 "Receive software fifo size:"; rcvmaxread4 "Receive maximum read:"; rcvminread4 "Receive minimum read:"; rcvusedelim4 "Read to delimiter:"; rcvdelim4 "Delimiter:"; rcvdatatype4 "Receive data type:"; rcvsampletime4 "Receive SampleTime:"
      mask help:
      | QSC-100
      | Quatech
      | RS232 Send Receive Subsystem
      mask init:
      | brdslot = slot;
      | mquamask( 1, 4 );
      mask Help: helpview(fullfile(docroot, 'mapfiles', 'xpc.map'), 'Quatech_Subsystem')
      mask StyleString: popup(Board Setup|Basic Setup|Transmit Setup|Receive Setup),popup(1|2|3|4),edit,edit,popup(921600|460800|230400|115200|57600|38400|19200|9600|4800|2400|1200|600|300|110),popup(None|Even|Odd|Mark|Space),popup(5|6|7|8),popup(1|2),popup(64 deep|16 deep|1 deep),popup(1|quarter full|half full|almost full),checkbox,edit,popup(count+32 bit int|count+32 bit uint|count+16 bit int|count+16 bit uint|8 bit int null terminated|8 bit uint null terminated),edit,edit,edit,checkbox,edit,popup(count+32 bit int|count+32 bit uint|count+16 bit int|count+16 bit uint|8 bit int null terminated|8 bit uint null terminated),edit,popup(921600|460800|230400|115200|57600|38400|19200|9600|4800|2400|1200|600|300|110),popup(None|Even|Odd|Mark|Space),popup(5|6|7|8),popup(1|2),popup(64 deep|16 deep|1 deep),popup(1|quarter full|half full|almost full),checkbox,edit,popup(count+32 bit int|count+32 bit uint|count+16 bit int|count+16 bit uint|8 bit int null terminated|8 bit uint null terminated),edit,edit,edit,checkbox,edit,popup(count+32 bit int|count+32 bit uint|count+16 bit int|count+16 bit uint|8 bit int null terminated|8 bit uint null terminated),edit,popup(921600|460800|230400|115200|57600|38400|19200|9600|4800|2400|1200|600|300|110),popup(None|Even|Odd|Mark|Space),popup(5|6|7|8),popup(1|2),popup(64 deep|16 deep|1 deep),popup(1|quarter full|half full|almost full),checkbox,edit,popup(count+32 bit int|count+32 bit uint|count+16 bit int|count+16 bit uint|8 bit int null terminated|8 bit uint null terminated),edit,edit,edit,checkbox,edit,popup(count+32 bit int|count+32 bit uint|count+16 bit int|count+16 bit uint|8 bit int null terminated|8 bit uint null terminated),edit,popup(921600|460800|230400|115200|57600|38400|19200|9600|4800|2400|1200|600|300|110),popup(None|Even|Odd|Mark|Space),popup(5|6|7|8),popup(1|2),popup(64 deep|16 deep|1 deep),popup(1|quarter full|half full|almost full),checkbox,edit,popup(count+32 bit int|count+32 bit uint|count+16 bit int|count+16 bit uint|8 bit int null terminated|8 bit uint null terminated),edit,edit,edit,checkbox,edit,popup(count+32 bit int|count+32 bit uint|count+16 bit int|count+16 bit uint|8 bit int null terminated|8 bit uint null terminated),edit
      mask CallbackString:
      | mquamask( 2, 4 );
      | |mquamask( 2, 4 );||||||||||||||||||||||||||||||||||||||||||||||||||||||||||||||||||
      mask Display:
      | disp('QSC-100\n\nRS232\n\nSend Receive');
      | port_label( 'input', 1, 'XMT1' );
      | port_label( 'input', 2, 'XMT2' );
      | port_label( 'input', 3, 'XMT3' );
      | port_label( 'input', 4, 'XMT4' );
      | port_label( 'output', 1, 'RCV1' );
      | port_label( 'output', 2, 'RCV2' );
      | port_label( 'output', 3, 'RCV3' );
      | port_label( 'output', 4, 'RCV4' );
  QSC-100 Internal  blocks : Subsystem
